simulink model "two_arm_keshe"  (R2025b)
settings: Solver=VariableStepAuto  StartTime=0.0  StopTime=2  RelTol=1e-3
settings Model: Creator=allen  LastModifiedBy=allen

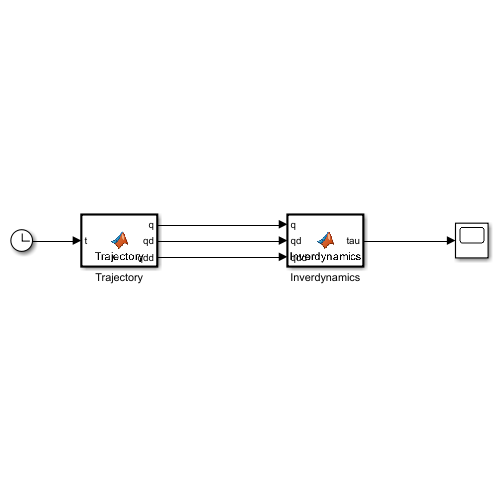
[thumbnail: Simulink's stored preview of the top-level diagram]
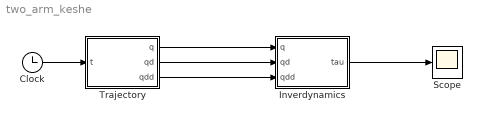
== system two_arm_keshe ==
  Clock : Clock
      settings: Decimation=100
  Inverdynamics : MATLAB Function  TreatAsAtomicUnit=on
  Scope : Scope
      settings: ActiveDisplayYMinimum=-608.327879645324  ActiveDisplayYMaximum=139.54153122714479
  Trajectory : MATLAB Function  TreatAsAtomicUnit=on
  wires:
  Inverdynamics/1(tau) -> Scope/1
  Trajectory/1(q) -> Inverdynamics/1(q)
  Trajectory/2(qd) -> Inverdynamics/2(qd)
  Trajectory/3(qdd) -> Inverdynamics/3(qdd)
  Clock/1 -> Trajectory/1(t)

== matlab function two_arm_keshe/Inverdynamics ==
  data: q input; tau output; qd input; qdd input
function tau = Inverdynamics(q, qd, qdd)
%% 动力学方程

%#codegen
% 调用外部函数计算逆动力学力矩
coder.extrinsic('computeTorque');

tau = zeros(1,6);              % 预分配，避免 coder 报错
tau = computeTorque(q, qd, qdd);
end

== matlab function two_arm_keshe/Trajectory ==
  data: q output; t input; qd output; qdd output
function [q, qd, qdd] = Trajectory(t)
%#codegen
% 五次多项式轨迹规划：从初始位形到目标位形
persistent q0 qf T

if isempty(q0)
    q0 = [0, 0, 0, 0, 0, 0];                          % 初始关节角
    qf = [pi/6, -pi/8, pi/4, pi/6, -pi/5, pi/3];      % 目标关节角
    T  = 2.0;                                          % 运动总时长 (s)
end

q   = zeros(1,6);
qd  = zeros(1,6);
qdd = zeros(1,6);

if t <= 0
    q = q0;
elseif t >= T
    q = qf;
else
    s   = t / T;
    s2  = s*s;  s3 = s2*s;  s4 = s3*s;  s5 = s4*s;
    h   = 10*s3 - 15*s4 + 6*s5;         % 位置插值函数
    hd  = 30*s2 - 60*s3 + 30*s4;        % 一阶导
    hdd = 60*s  - 180*s2 + 120*s3;      % 二阶导
    
    dq  = qf - q0;
    q   = q0 + dq * h;
    qd  = dq * hd  / T;
    qdd = dq * hdd / (T*T);
end
end
